simulink model "qubetemplate"  (R2021b)
settings: Solver=ode1  StartTime=0.0  StopTime=T  RelTol=1e-3  EnableMultiTasking=on
values from neighbouring files (symbols this model uses):
  h = 0.01    [Qubefile.m]    (also in calibration.m; runexp.m)
undefined symbols (not defined in the file or in its folder): Humusoft, MF634
libraries: sldrtlib x2
settings Model: Creator=rbabuska  LastModifiedBy=oscarhe
settings SolverCC: AlgebraicLoopSolver=TrustRegion
settings DataIOCC: LimitDataPoints=on  SaveFormat=Array  SignalLoggingSaveFormat=ModelDataLogs  ReturnWorkspaceOutputs=off
settings OptimizationCC: ExpressionDepthLimit=2147483647  LifeSpan=inf
settings DebuggingCC: UnderspecifiedInitializationDetection=Classic  MergeDetectMultiDrivingBlocksExec=none  FcnCallInpInsideContextMsg=warning  StateNameClashWarn=warning  SFUnexpectedBacktrackingDiag=warning  SFNoUnconditionalDefaultTransitionDiag=warning  SFExecutionAtInitializationDiag=none  SFMachineParentedDataDiag=warning  ArithmeticOperatorsInVariantConditions=warning
settings HardwareCC: ProdBitPerPointer=32  ProdBitPerSizeT=32  ProdBitPerPtrDiffT=32  ProdLargestAtomicFloat=None  ProdIntDivRoundTo=Undefined  ProdEndianess=Unspecified  ProdWordSize=32  ProdHWDeviceType=32-bit Generic
settings ModelReferenceCC: PropagateSignalLabelsOutOfModel=off
settings SFSimCC: SimUseLocalCustomCode=off  CustomCodeUndefinedFunction=UseInterfaceOnly
settings RTWCC: RTWUseLocalCustomCode=off
settings CodeAppCC: StateflowObjectComments=on
settings GRTTargetCC: TargetLangStandard=C89/C90 (ANSI)  CombineOutputUpdateFcns=off  GRTInterface=on
settings ConfigComp: CovMetricSettings=dw  CovSaveCumulativeToWorkspaceVar=on  CovSaveSingleToWorkspaceVar=on  CovExternalEMLEnable=off  CovSFcnEnable=off

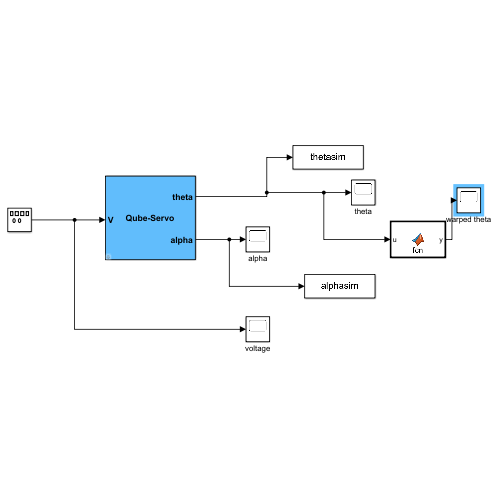
[thumbnail: Simulink's stored preview of the top-level diagram]
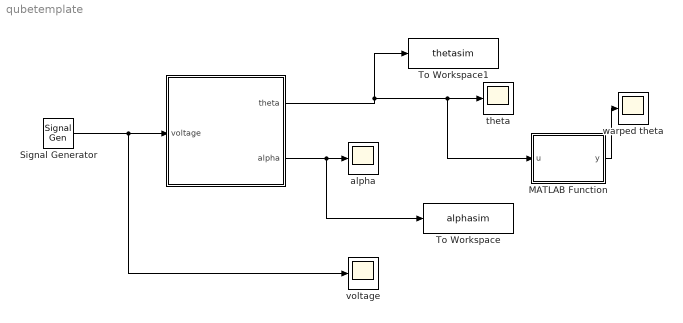
== system qubetemplate ==
  " " : Subsystem  LoadFcn=hwinit  InitFcn=hwinit  mask{h=h}
      mask prompts: h "Sampling period [s]"
      mask Display:
      | disp('Qube-Servo')
      | port_label('output',1,'theta')
      | port_label('output',2,'alpha')
      | port_label('input',1,'V')
  MATLAB Function : MATLAB Function  TreatAsAtomicUnit=on
  Signal Generator : SignalGenerator  Amplitude=0
  To Workspace : ToWorkspace  VariableName=alphasim  SaveFormat=Timeseries  SampleTime=-1
  To Workspace1 : ToWorkspace  VariableName=thetasim  SaveFormat=Timeseries  SampleTime=-1
  alpha : Scope
  theta : Scope
  voltage : Scope
  warped theta : Scope
  wires:
  Signal Generator/1 -> " "/1(voltage), voltage/1
  " "/1(theta) -> To Workspace1/1, MATLAB Function/1(u), theta/1
  " "/2(alpha) -> To Workspace/1, alpha/1
  MATLAB Function/1(y) -> warped theta/1

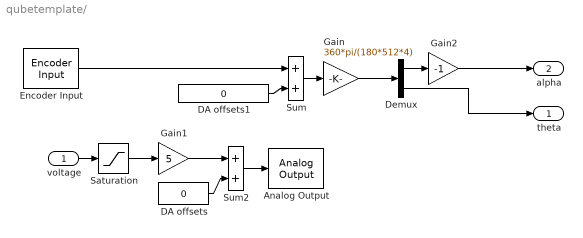
== system qubetemplate/  ==
  voltage : Inport
  Analog Output : sldrtlib/Analog Output  SampleTime=h  MaxMissedTicks=100  ShowMissedTicks=off  YieldWhenWaiting=off  DrvName=Humusoft/MF634  DrvAddress=4294967295  DrvOptions=0  Channels=[1]  RangeMode=2  VoltRange=1  InitialValue=0  FinalValue=0
      settings: AttributesFormatString=Humusoft\nMF634 [auto]
  DA offsets : Constant  Value=0
  DA offsets1 : Constant  Value=0  SampleTime=h
  Demux : Demux  Outputs=2
  Encoder Input : sldrtlib/Encoder Input  SampleTime=h  MaxMissedTicks=100  ShowMissedTicks=off  YieldWhenWaiting=off  DrvName=Humusoft/MF634  DrvAddress=4294967295  DrvOptions=0  Channels=[1,2]  QuadMode=3  IndexPulse=1  InputFilter=Inf  DataType=1
      settings: AttributesFormatString=Humusoft\nMF634 [auto]
  Gain : Gain  Gain=360*pi/(180*512*4)  SaturateOnIntegerOverflow=on  OutDataTypeStr=Inherit: Same as input  ParamDataTypeStr=Inherit: Same as input
  Gain1 : Gain  Gain=5  SaturateOnIntegerOverflow=on  OutDataTypeStr=Inherit: Same as input  ParamDataTypeStr=Inherit: Same as input
  Gain2 : Gain  Gain=-1  SaturateOnIntegerOverflow=on  OutDataTypeStr=Inherit: Same as input  ParamDataTypeStr=Inherit: Same as input
  Saturation : Saturate  UpperLimit=1  LowerLimit=-1
  Sum : Sum  InputSameDT=on  SaturateOnIntegerOverflow=on  OutDataTypeStr=Inherit: Same as first input
  Sum2 : Sum  InputSameDT=on  SaturateOnIntegerOverflow=on  OutDataTypeStr=Inherit: Same as first input
  theta : Outport  Tag=Cable length
  alpha : Outport  Tag=Cable length  Port=2
  wires:
  Sum/1 -> Gain/1
  DA offsets1/1 -> Sum/2
  Gain1/1 -> Sum2/1
  Sum2/1 -> Analog Output/1
  DA offsets/1 -> Sum2/2
  voltage/1 -> Saturation/1
  Encoder Input/1 -> Sum/1
  Saturation/1 -> Gain1/1
  Demux/1 -> Gain2/1
  Gain/1 -> Demux/1
  Gain2/1 -> alpha/1
  Demux/2 -> theta/1

== matlab function qubetemplate/MATLAB Function ==
  data: u input; y output
function y = fcn(u)


y = u - 2*pi*floor((u+pi)/(2*pi));
